simulink library "dgl_grc"  (R2024a)
settings: Solver=VariableStepAuto  StartTime=0.0  StopTime=10.0  RelTol=1e-3
undefined symbols (not defined in the file or in its folder): Diag2_bRstFault_C, Diag2_f32_UdcLowCoefAddStep_C, Diag2_f32_UdcLowCoefDepStep_C, Diag2_f32_UdcLowHysBand_C, Diag2_f32_UdcLowStartDerat_C, Diag2_f32_UdcLowStopDerat_C, Diag2_f32_UdcOverCoefAddStep_C, Diag2_f32_UdcOverCoefDepStep_C, Diag2_f32_UdcOverHysBand_C, Diag2_f32_UdcOverStartDerat_C, Diag2_f32_UdcOverStopDerat_C, Diag2_int16_HvLowErrErr_C, Diag2_int16_HvLowErrHeal_C, Diag2_int16_HvLowWarnErr_C, Diag2_int16_HvLowWarnHeal_C, Diag2_int16_HvOverErrErr_C, Diag2_int16_HvOverErrHeal_C, Diag2_int16_HvOverWarnErr_C, Diag2_int16_HvOverWarnHeal_C, DiagM_bZeroCurrMor_C, DiagM_bZeroCurrTrig_C, DiagM_Fault2LevelMor_C, DiagM_Fault2LevelTrig_C, GRC_FAKE_SAMPLE_TIME, KDGL_bBusOffEna_C, KDGL_bComInvaildVcuEna_C, KDGL_bComLostVcuEna_C, KDGL_bCurrFaultEna_C, KDGL_bEnaBenchShutDwn_C, KDGL_bEOPFaultEna_C, KDGL_bHvDcVoltFaultEna_C, KDGL_bIGNVoltFaultEna_C, KDGL_bOilTempFaultEna_C, KDGL_bPCBTempFaultEna_C, KDGL_bPosSenrFaultEna_C, KDGL_bPREREGFaultEna_C, KDGL_bRstStallPort_flg, KDGL_bSicFltFaultEna_C, KDGL_bSicTempFaultEna_C, KDGL_bTempSensrFaultEna_C, KDGL_bVCC5VFaultEna_C, KDGL_bVREF5VFaultEna_C, KDGL_bWaterTempFaultEna_C, KDGL_IGBTCoefAddStep_C, KDGL_IGBTCoefDepStep_C, KDGL_IGBTHysBand_C, KDGL_IGBTStartDerat_C, KDGL_IGBTStopDerat_C, KDGL_iMotStallProtEna_A, KDGL_MotCoefAddStep_C, KDGL_MotCoefDepStep_C, KDGL_MotHysBand_C, KDGL_MotStartDerat_C, KDGL_MotStopDerat_C, KDGL_nEOPSpdDiff_rpm, KDGL_nRotStallProtEna_rpm, KDGL_OilCoefAddStep_C, KDGL_OilCoefDepStep_C, KDGL_OilHysBand_C, KDGL_OilStartDerat_C ... (+37)
libraries: Library x28, GRC_Lib x8
(part 2 of 2)

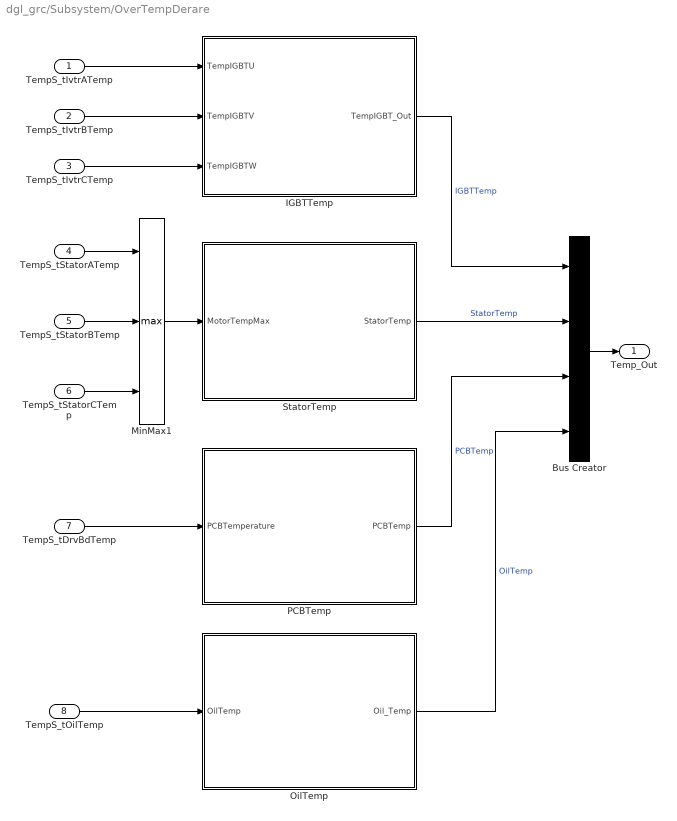
== system dgl_grc/Subsystem/OverTempDerare ==
  TempS_tIvtrATemp : Inport  OutDataTypeStr=single
  TempS_tIvtrBTemp : Inport  Port=2  OutDataTypeStr=single
  TempS_tIvtrCTemp : Inport  Port=3  OutDataTypeStr=single
  TempS_tStatorATemp : Inport  Port=4  OutDataTypeStr=single
  TempS_tStatorBTemp : Inport  Port=5  OutDataTypeStr=single
  TempS_tStatorCTemp : Inport  Port=6  OutDataTypeStr=single
  TempS_tDrvBdTemp : Inport  Port=7  OutDataTypeStr=single
  TempS_tOilTemp : Inport  Port=8  OutDataTypeStr=single
  Bus Creator : BusCreator  Inputs=4
  IGBTTemp : Subsystem
  MinMax1 : MinMax  Function=max  Inputs=3
  OilTemp : Subsystem
  PCBTemp : Subsystem
  StatorTemp : Subsystem
  Temp_Out : Outport  VectorParamsAs1DForOutWhenUnconnected=off
  wires:
  TempS_tIvtrATemp/1 -> IGBTTemp/1(TempIGBTU)
  TempS_tIvtrBTemp/1 -> IGBTTemp/2(TempIGBTV)
  TempS_tIvtrCTemp/1 -> IGBTTemp/3(TempIGBTW)
  TempS_tStatorBTemp/1 -> MinMax1/2
  TempS_tStatorATemp/1 -> MinMax1/1
  TempS_tStatorCTemp/1 -> MinMax1/3
  MinMax1/1 -> StatorTemp/1(MotorTempMax)
  TempS_tDrvBdTemp/1 -> PCBTemp/1(PCBTemperature)
  StatorTemp/1(StatorTemp) -> Bus Creator/2  "StatorTemp"
  IGBTTemp/1(TempIGBT_Out) -> Bus Creator/1  "IGBTTemp"
  PCBTemp/1(PCBTemp) -> Bus Creator/3  "PCBTemp"
  Bus Creator/1 -> Temp_Out/1
  TempS_tOilTemp/1 -> OilTemp/1(OilTemp)
  OilTemp/1(Oil_Temp) -> Bus Creator/4  "OilTemp"

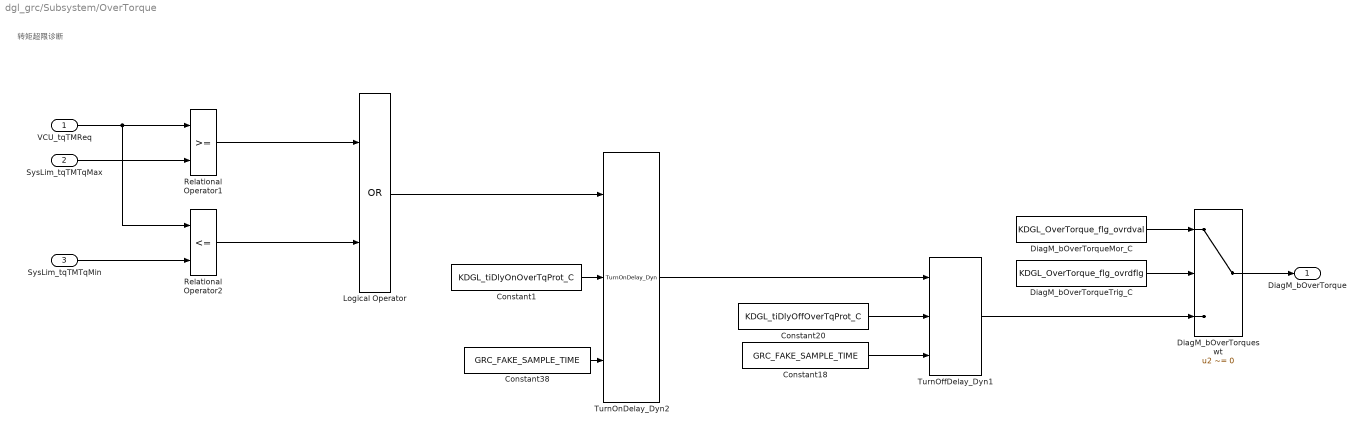
== system dgl_grc/Subsystem/OverTorque ==
  note: 转矩超限诊断
  VCU_tqTMReq : Inport  OutDataTypeStr=single
  SysLim_tqTMTqMax : Inport  Port=2  OutDataTypeStr=single
  "SysLim_tqTMTqMin " : Inport  Port=3  OutDataTypeStr=single
  Constant1 : Constant  Value=KDGL_tiDlyOnOverTqProt_C
  Constant18 : Constant  Value=GRC_FAKE_SAMPLE_TIME
  Constant20 : Constant  Value=KDGL_tiDlyOffOverTqProt_C
  Constant38 : Constant  Value=GRC_FAKE_SAMPLE_TIME
  DiagM_bOverTorqueMor_C : Constant  Value=KDGL_OverTorque_flg_ovrdval
  DiagM_bOverTorqueTrig_C : Constant  Value=KDGL_OverTorque_flg_ovrdflg
  DiagM_bOverTorqueswt : Switch  Criteria=u2 ~= 0  SaturateOnIntegerOverflow=off  InputSameDT=off
  Logical Operator : Logic  Operator=OR  AllPortsSameDT=off  OutDataTypeStr=boolean
  Relational Operator1 : RelationalOperator  OutDataTypeStr=boolean  RndMeth=Simplest  InputSameDT=off
  Relational Operator2 : RelationalOperator  Operator=<=  OutDataTypeStr=boolean  RndMeth=Simplest  InputSameDT=off
  TurnOffDelay_Dyn1 : GRC_Lib/Delay/TurnOffDelay_Dyn  IpDT=single
  TurnOnDelay_Dyn2 : GRC_Lib/Delay/TurnOnDelay_Dyn  IpDT=single
  DiagM_bOverTorque : Outport  VectorParamsAs1DForOutWhenUnconnected=off
  wires:
  Constant1/1 -> TurnOnDelay_Dyn2/2
  VCU_tqTMReq/1 -> Relational Operator2/1, Relational Operator1/1
  TurnOnDelay_Dyn2/1 -> TurnOffDelay_Dyn1/1
  Constant38/1 -> TurnOnDelay_Dyn2/3
  Constant18/1 -> TurnOffDelay_Dyn1/3
  TurnOffDelay_Dyn1/1 -> DiagM_bOverTorqueswt/3
  Constant20/1 -> TurnOffDelay_Dyn1/2
  Relational Operator1/1 -> Logical Operator/1
  SysLim_tqTMTqMax/1 -> Relational Operator1/2
  "SysLim_tqTMTqMin "/1 -> Relational Operator2/2
  Relational Operator2/1 -> Logical Operator/2
  Logical Operator/1 -> TurnOnDelay_Dyn2/1
  DiagM_bOverTorqueswt/1 -> DiagM_bOverTorque/1
  DiagM_bOverTorqueMor_C/1 -> DiagM_bOverTorqueswt/1
  DiagM_bOverTorqueTrig_C/1 -> DiagM_bOverTorqueswt/2

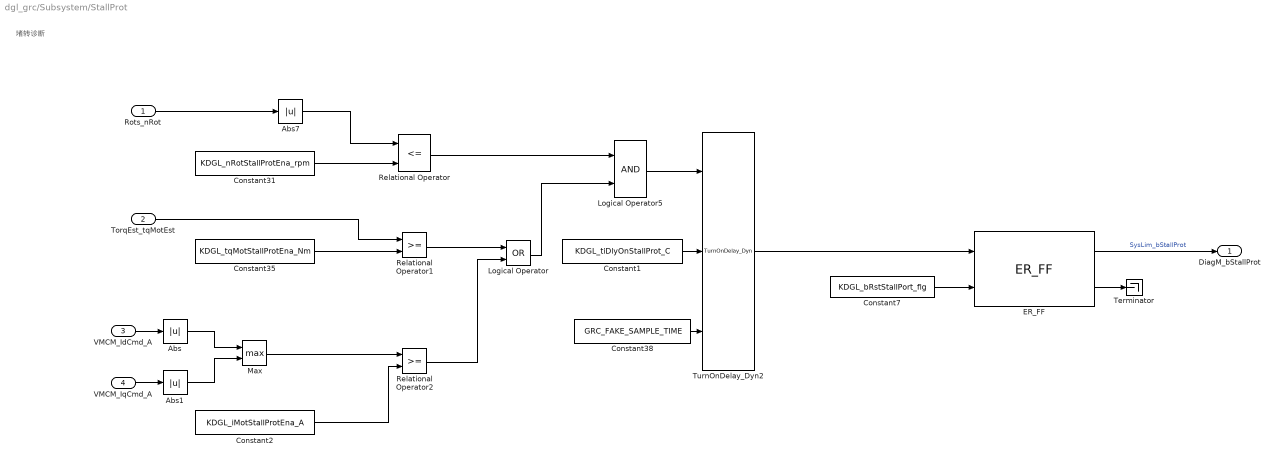
== system dgl_grc/Subsystem/StallProt ==
  note: 堵转诊断
  Rots_nRot : Inport  OutDataTypeStr=single
  TorqEst_tqMotEst : Inport  Port=2  OutDataTypeStr=single
  VMCM_IdCmd_A : Inport  Port=3  OutDataTypeStr=single
  VMCM_IqCmd_A : Inport  Port=4  OutDataTypeStr=single
  Abs : Abs  SaturateOnIntegerOverflow=off
  Abs1 : Abs  SaturateOnIntegerOverflow=off
  Abs7 : Abs  SaturateOnIntegerOverflow=off
  Constant1 : Constant  Value=KDGL_tiDlyOnStallProt_C
  Constant2 : Constant  Value=KDGL_iMotStallProtEna_A
  Constant31 : Constant  Value=KDGL_nRotStallProtEna_rpm
  Constant35 : Constant  Value=KDGL_tqMotStallProtEna_Nm
  Constant38 : Constant  Value=GRC_FAKE_SAMPLE_TIME
  Constant7 : Constant  Value=KDGL_bRstStallPort_flg
  ER_FF : GRC_Lib/Memory/ER_FF  FalseVal=0  TrueVal=1
  Logical Operator : Logic  Operator=OR  AllPortsSameDT=off  OutDataTypeStr=boolean
  Logical Operator5 : Logic  AllPortsSameDT=off  OutDataTypeStr=boolean
  Max : MinMax  Function=max  Inputs=2
  Relational Operator : RelationalOperator  Operator=<=  OutDataTypeStr=boolean  RndMeth=Simplest  InputSameDT=off
  Relational Operator1 : RelationalOperator  OutDataTypeStr=boolean  RndMeth=Simplest  InputSameDT=off
  Relational Operator2 : RelationalOperator  OutDataTypeStr=boolean  RndMeth=Simplest  InputSameDT=off
  Terminator : Terminator
  TurnOnDelay_Dyn2 : GRC_Lib/Delay/TurnOnDelay_Dyn  IpDT=single
  DiagM_bStallProt : Outport  VectorParamsAs1DForOutWhenUnconnected=off
  wires:
  ER_FF/1 -> DiagM_bStallProt/1  "SysLim_bStallProt"
  Abs7/1 -> Relational Operator/1
  Rots_nRot/1 -> Abs7/1
  Logical Operator5/1 -> TurnOnDelay_Dyn2/1
  Constant35/1 -> Relational Operator1/2
  Relational Operator/1 -> Logical Operator5/1
  Relational Operator1/1 -> Logical Operator/1
  Constant38/1 -> TurnOnDelay_Dyn2/3
  Constant31/1 -> Relational Operator/2
  TorqEst_tqMotEst/1 -> Relational Operator1/1
  Constant1/1 -> TurnOnDelay_Dyn2/2
  TurnOnDelay_Dyn2/1 -> ER_FF/1
  Constant7/1 -> ER_FF/2
  ER_FF/2 -> Terminator/1
  VMCM_IdCmd_A/1 -> Abs/1
  VMCM_IqCmd_A/1 -> Abs1/1
  Abs/1 -> Max/1
  Abs1/1 -> Max/2
  Max/1 -> Relational Operator2/1
  Constant2/1 -> Relational Operator2/2
  Relational Operator2/1 -> Logical Operator/2
  Logical Operator/1 -> Logical Operator5/2

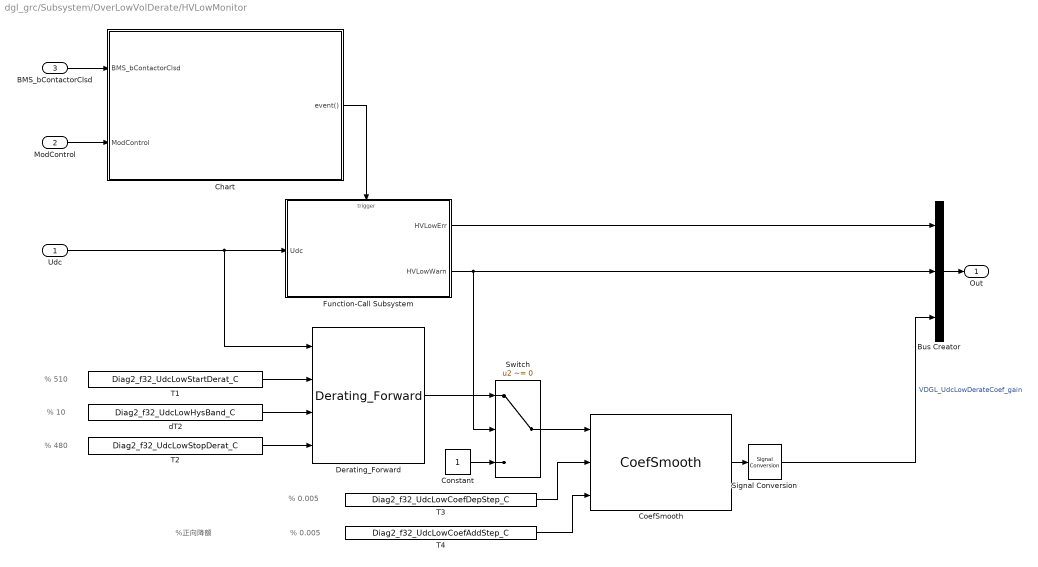
== system dgl_grc/Subsystem/OverLowVolDerate/HVLowMonitor ==
  note: % 510
  note: % 0.005
  note: %正向降额
  note: % 0.005
  note: % 480
  note: % 10
  Udc : Inport
  ModControl : Inport  Port=2
  BMS_bContactorClsd : Inport  Port=3
  Bus Creator : BusCreator  Inputs=3
  Chart : Stateflow chart  TreatAsAtomicUnit=on
  CoefSmooth : Library/CoefSmooth  SystemSampleTime=-1  VariantActivationTime=update diagram  AllowFlexibleInterface=on  Latency=0  AutoFrameSizeCalculation=off
  Constant : Constant  OutDataTypeStr=single
  Derating_Forward : Library/Derating_Forward  SystemSampleTime=-1  VariantActivationTime=update diagram  AllowFlexibleInterface=on  Latency=0  AutoFrameSizeCalculation=off
  Function-Call Subsystem : Subsystem  TreatAsAtomicUnit=on
  Signal Conversion : SignalConversion  OverrideOpt=off
  Switch : Switch  Criteria=u2 ~= 0  SaturateOnIntegerOverflow=off  InputSameDT=off
  T1 : Constant  Value=Diag2_f32_UdcLowStartDerat_C  OutDataTypeStr=single
  T2 : Constant  Value=Diag2_f32_UdcLowStopDerat_C  OutDataTypeStr=single
  T3 : Constant  Value=Diag2_f32_UdcLowCoefDepStep_C  OutDataTypeStr=single
  T4 : Constant  Value=Diag2_f32_UdcLowCoefAddStep_C  OutDataTypeStr=single
  dT2 : Constant  Value=Diag2_f32_UdcLowHysBand_C  OutDataTypeStr=single
  Out : Outport  VectorParamsAs1DForOutWhenUnconnected=off
  wires:
  Chart/1(event()) -> Function-Call Subsystem/Trigger
  Function-Call Subsystem/1(HVLowErr) -> Bus Creator/1
  Bus Creator/1 -> Out/1
  Function-Call Subsystem/2(HVLowWarn) -> Switch/2, Bus Creator/2
  dT2/1 -> Derating_Forward/3
  T1/1 -> Derating_Forward/2
  T2/1 -> Derating_Forward/4
  Derating_Forward/1 -> Switch/1
  Constant/1 -> Switch/3
  Switch/1 -> CoefSmooth/1
  T3/1 -> CoefSmooth/2
  T4/1 -> CoefSmooth/3
  CoefSmooth/1 -> Signal Conversion/1
  Signal Conversion/1 -> Bus Creator/3  "VDGL_UdcLowDerateCoef_gain"
  ModControl/1 -> Chart/2(ModControl)
  Udc/1 -> Derating_Forward/1, Function-Call Subsystem/1(Udc)
  BMS_bContactorClsd/1 -> Chart/1(BMS_bContactorClsd)

== system dgl_grc/Subsystem/OverLowVolDerate/HVOverMonitor ==
  note: 反向降额
  note: % 20
  note: % 880
  note: % 750
  note: % 0.005
  note: % 0.005
  Udc : Inport
  Bus Creator : BusCreator  Inputs=3
  CoefSmooth : Library/CoefSmooth  SystemSampleTime=-1  VariantActivationTime=update diagram  AllowFlexibleInterface=on  Latency=0  AutoFrameSizeCalculation=off
  Constant : Constant  OutDataTypeStr=single
  Derating_Reverse : Library/Derating_Reverse  SystemSampleTime=-1  VariantActivationTime=update diagram  AllowFlexibleInterface=on  Latency=0  AutoFrameSizeCalculation=off
  Function-Call Subsystem : Subsystem  TreatAsAtomicUnit=on
  Signal Conversion : SignalConversion  OverrideOpt=off
  Switch : Switch  Criteria=u2 ~= 0  SaturateOnIntegerOverflow=off  InputSameDT=off
  T1 : Constant  Value=Diag2_f32_UdcOverStartDerat_C  OutDataTypeStr=single
  T2 : Constant  Value=Diag2_f32_UdcOverStopDerat_C  OutDataTypeStr=single
  T3 : Constant  Value=Diag2_f32_UdcOverCoefDepStep_C  OutDataTypeStr=single
  T4 : Constant  Value=Diag2_f32_UdcOverCoefAddStep_C  OutDataTypeStr=single
  dT2 : Constant  Value=Diag2_f32_UdcOverHysBand_C  OutDataTypeStr=single
  Out : Outport  VectorParamsAs1DForOutWhenUnconnected=off
  wires:
  Udc/1 -> Derating_Reverse/1, Function-Call Subsystem/1(Udc)
  Bus Creator/1 -> Out/1
  Function-Call Subsystem/2(HVOverWarn) -> Switch/2, Bus Creator/2
  Function-Call Subsystem/1(HVOverErr) -> Bus Creator/1
  dT2/1 -> Derating_Reverse/3
  T1/1 -> Derating_Reverse/2
  T2/1 -> Derating_Reverse/4
  Derating_Reverse/1 -> Switch/1
  Constant/1 -> Switch/3
  Switch/1 -> CoefSmooth/1
  T3/1 -> CoefSmooth/2
  T4/1 -> CoefSmooth/3
  CoefSmooth/1 -> Signal Conversion/1
  Signal Conversion/1 -> Bus Creator/3  "VDGL_UdcOverDerateCoef_gain"

== system dgl_grc/Subsystem/OverSpdDerate/Function-Call Subsystem ==
  note: % 20
  note: % -20
  note: % 1000
  note: % 22000
  note: %速度滞环
  MeclSpd : Inport
  Constant : Constant  Value=KDGL_OverSpd_rpm  OutDataTypeStr=single
  Constant1 : Constant  Value=KDGL_OverSpdHeal_cnt  OutDataTypeStr=int16
  Constant2 : Constant  Value=KDGL_OverSpdErr_cnt  OutDataTypeStr=int16
  Constant3 : Constant  Value=KDGL_OverSpdHysBand_rpm  OutDataTypeStr=single
  Hysteresis_Ctrl_Forward : Library/Hysteresis_Ctrl_Forward  SystemSampleTime=-1  VariantActivationTime=update diagram  AllowFlexibleInterface=on  Latency=0  AutoFrameSizeCalculation=off
  Signal Conversion : SignalConversion  OverrideOpt=off
  debounce : Library/debounce  SystemSampleTime=-1  VariantActivationTime=update diagram  AllowFlexibleInterface=on  Latency=0  AutoFrameSizeCalculation=off
  OverSpdFlg : Outport  VectorParamsAs1DForOutWhenUnconnected=off
  wires:
  Constant1/1 -> debounce/2
  Constant2/1 -> debounce/3
  Signal Conversion/1 -> OverSpdFlg/1
  debounce/1 -> Signal Conversion/1
  Constant/1 -> Hysteresis_Ctrl_Forward/2
  Constant3/1 -> Hysteresis_Ctrl_Forward/3
  Hysteresis_Ctrl_Forward/1 -> debounce/1
  MeclSpd/1 -> Hysteresis_Ctrl_Forward/1

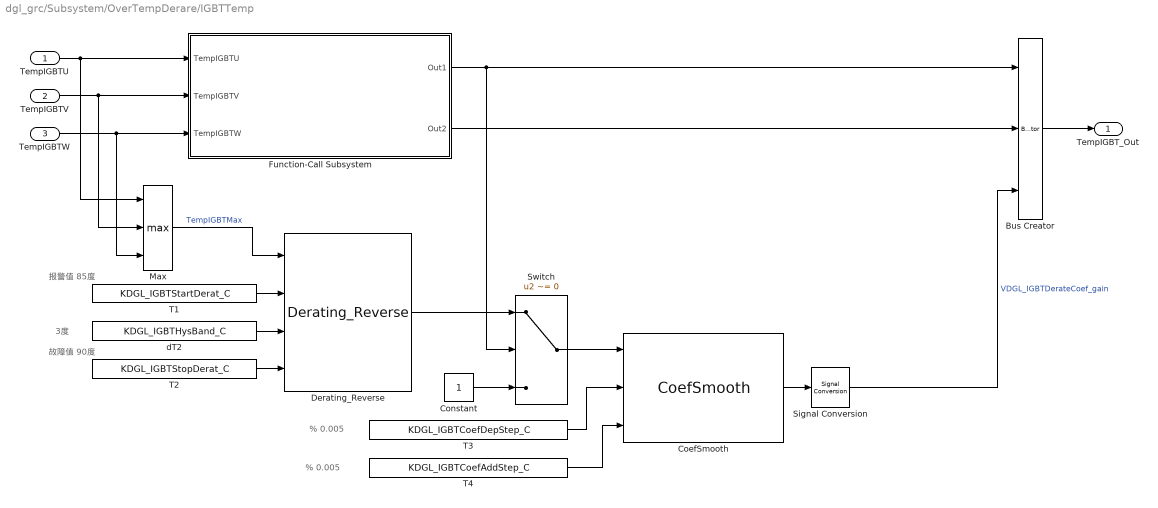
== system dgl_grc/Subsystem/OverTempDerare/IGBTTemp ==
  note: % 0.005
  note: 报警值
      | 85度
  note: 3度
  note: 故障值
      | 90度
  note: % 0.005
  TempIGBTU : Inport
  TempIGBTV : Inport  Port=2
  TempIGBTW : Inport  Port=3
  Bus Creator : BusCreator  Inputs=3
  CoefSmooth : Library/CoefSmooth  SystemSampleTime=-1  VariantActivationTime=update diagram  AllowFlexibleInterface=on  Latency=0  AutoFrameSizeCalculation=off
  Constant : Constant  OutDataTypeStr=single
  Derating_Reverse : Library/Derating_Reverse  SystemSampleTime=-1  VariantActivationTime=update diagram  AllowFlexibleInterface=on  Latency=0  AutoFrameSizeCalculation=off
  Function-Call Subsystem : Subsystem  TreatAsAtomicUnit=on
  Max : MinMax  Function=max  Inputs=3
  Signal Conversion : SignalConversion  OverrideOpt=off
  Switch : Switch  Criteria=u2 ~= 0  SaturateOnIntegerOverflow=off  InputSameDT=off
  T1 : Constant  Value=KDGL_IGBTStartDerat_C  OutDataTypeStr=single
  T2 : Constant  Value=KDGL_IGBTStopDerat_C  OutDataTypeStr=single
  T3 : Constant  Value=KDGL_IGBTCoefDepStep_C  OutDataTypeStr=single
  T4 : Constant  Value=KDGL_IGBTCoefAddStep_C  OutDataTypeStr=single
  dT2 : Constant  Value=KDGL_IGBTHysBand_C  OutDataTypeStr=single
  TempIGBT_Out : Outport  VectorParamsAs1DForOutWhenUnconnected=off
  wires:
  Bus Creator/1 -> TempIGBT_Out/1
  Function-Call Subsystem/1(Out1) -> Switch/2, Bus Creator/1
  Function-Call Subsystem/2(Out2) -> Bus Creator/2
  dT2/1 -> Derating_Reverse/3
  T1/1 -> Derating_Reverse/2
  T2/1 -> Derating_Reverse/4
  Derating_Reverse/1 -> Switch/1
  Constant/1 -> Switch/3
  Switch/1 -> CoefSmooth/1
  T3/1 -> CoefSmooth/2
  T4/1 -> CoefSmooth/3
  CoefSmooth/1 -> Signal Conversion/1
  Signal Conversion/1 -> Bus Creator/3  "VDGL_IGBTDerateCoef_gain"
  TempIGBTU/1 -> Max/1, Function-Call Subsystem/1(TempIGBTU)
  TempIGBTV/1 -> Max/2, Function-Call Subsystem/2(TempIGBTV)
  TempIGBTW/1 -> Max/3, Function-Call Subsystem/3(TempIGBTW)
  Max/1 -> Derating_Reverse/1  "TempIGBTMax"

== system dgl_grc/Subsystem/OverTempDerare/OilTemp ==
  note: % 0.005
  note: 报警值
      | 110度
  note: 3度
  note: 故障值
      | 120度
  note: % 0.005
  OilTemp : Inport
  Bus Creator : BusCreator  Inputs=3
  CoefSmooth : Library/CoefSmooth  SystemSampleTime=-1  VariantActivationTime=update diagram  AllowFlexibleInterface=on  Latency=0  AutoFrameSizeCalculation=off
  Constant : Constant  OutDataTypeStr=single
  Derating_Reverse : Library/Derating_Reverse  SystemSampleTime=-1  VariantActivationTime=update diagram  AllowFlexibleInterface=on  Latency=0  AutoFrameSizeCalculation=off
  Function-Call Subsystem : Subsystem  TreatAsAtomicUnit=on
  Signal Conversion : SignalConversion  OverrideOpt=off
  Switch : Switch  Criteria=u2 ~= 0  SaturateOnIntegerOverflow=off  InputSameDT=off
  T1 : Constant  Value=KDGL_OilStartDerat_C  OutDataTypeStr=single
  T2 : Constant  Value=KDGL_OilStopDerat_C  OutDataTypeStr=single
  T3 : Constant  Value=KDGL_OilCoefDepStep_C  OutDataTypeStr=single
  T4 : Constant  Value=KDGL_OilCoefAddStep_C  OutDataTypeStr=single
  dT2 : Constant  Value=KDGL_OilHysBand_C  OutDataTypeStr=single
  Oil_Temp : Outport  VectorParamsAs1DForOutWhenUnconnected=off
  wires:
  Bus Creator/1 -> Oil_Temp/1
  Function-Call Subsystem/2(Out1) -> Bus Creator/2
  Function-Call Subsystem/1(Out) -> Switch/2, Bus Creator/1
  dT2/1 -> Derating_Reverse/3
  T1/1 -> Derating_Reverse/2
  T2/1 -> Derating_Reverse/4
  Derating_Reverse/1 -> Switch/1
  Constant/1 -> Switch/3
  Switch/1 -> CoefSmooth/1
  T3/1 -> CoefSmooth/2
  T4/1 -> CoefSmooth/3
  CoefSmooth/1 -> Signal Conversion/1
  Signal Conversion/1 -> Bus Creator/3  "VDGL_OilDerateCoef_gain"
  OilTemp/1 -> Derating_Reverse/1, Function-Call Subsystem/1(OilTemp)

== system dgl_grc/Subsystem/OverTempDerare/PCBTemp ==
  note: 报警值
      | 85度
  note: 3度
  note: 故障值
      | 90度
  note: % 0.005
  note: % 0.005
  PCBTemperature : Inport
  Bus Creator : BusCreator  Inputs=3
  CoefSmooth : Library/CoefSmooth  SystemSampleTime=-1  VariantActivationTime=update diagram  AllowFlexibleInterface=on  Latency=0  AutoFrameSizeCalculation=off
  Constant : Constant  OutDataTypeStr=single
  Derating_Reverse : Library/Derating_Reverse  SystemSampleTime=-1  VariantActivationTime=update diagram  AllowFlexibleInterface=on  Latency=0  AutoFrameSizeCalculation=off
  Function-Call Subsystem : Subsystem  TreatAsAtomicUnit=on
  Signal Conversion : SignalConversion  OverrideOpt=off
  Switch : Switch  Criteria=u2 ~= 0  SaturateOnIntegerOverflow=off  InputSameDT=off
  T1 : Constant  Value=KDGL_PCBStartDerat_C  OutDataTypeStr=single
  T2 : Constant  Value=KDGL_PCBStopDerat_C  OutDataTypeStr=single
  T3 : Constant  Value=KDGL_PCBCoefDepStep_C  OutDataTypeStr=single
  T4 : Constant  Value=KDGL_PCBCoefAddStep_C  OutDataTypeStr=single
  dT2 : Constant  Value=KDGL_PCBHysBand_C  OutDataTypeStr=single
  PCBTemp : Outport  VectorParamsAs1DForOutWhenUnconnected=off
  wires:
  Bus Creator/1 -> PCBTemp/1
  Function-Call Subsystem/2(Out1) -> Bus Creator/2
  Function-Call Subsystem/1(Out) -> Switch/2, Bus Creator/1
  dT2/1 -> Derating_Reverse/3
  T1/1 -> Derating_Reverse/2
  T2/1 -> Derating_Reverse/4
  Derating_Reverse/1 -> Switch/1
  Constant/1 -> Switch/3
  Switch/1 -> CoefSmooth/1
  T3/1 -> CoefSmooth/2
  T4/1 -> CoefSmooth/3
  CoefSmooth/1 -> Signal Conversion/1
  Signal Conversion/1 -> Bus Creator/3  "VDGL_PCBDerateCoef_gain"
  PCBTemperature/1 -> Derating_Reverse/1, Function-Call Subsystem/1(PCBTemp)

== system dgl_grc/Subsystem/OverTempDerare/StatorTemp ==
  note: 10度
  note: 故障值
      | 120度
  note: 报警值
      | 110度
  note: % 0.005
  note: % 0.005
  MotorTempMax : Inport
  Bus Creator : BusCreator  Inputs=3
  CoefSmooth : Library/CoefSmooth  SystemSampleTime=-1  VariantActivationTime=update diagram  AllowFlexibleInterface=on  Latency=0  AutoFrameSizeCalculation=off
  Constant : Constant  OutDataTypeStr=single
  Function-Call Subsystem : Subsystem  TreatAsAtomicUnit=on
  Signal Conversion : SignalConversion  OverrideOpt=off
  Switch : Switch  Criteria=u2 ~= 0  SaturateOnIntegerOverflow=off  InputSameDT=off
  T3 : Constant  Value=KDGL_MotStartDerat_C  OutDataTypeStr=single
  T4 : Constant  Value=KDGL_MotStopDerat_C  OutDataTypeStr=single
  T5 : Constant  Value=KDGL_MotCoefDepStep_C  OutDataTypeStr=single
  T6 : Constant  Value=KDGL_MotCoefAddStep_C  OutDataTypeStr=single
  Temp_Derating_Reverse : Library/Derating_Reverse  SystemSampleTime=-1  VariantActivationTime=update diagram  AllowFlexibleInterface=on  Latency=0  AutoFrameSizeCalculation=off
  dT1 : Constant  Value=KDGL_MotHysBand_C  OutDataTypeStr=single
  StatorTemp : Outport  VectorParamsAs1DForOutWhenUnconnected=off
  wires:
  MotorTempMax/1 -> Temp_Derating_Reverse/1, Function-Call Subsystem/1(MotorTemp)
  Bus Creator/1 -> StatorTemp/1
  Function-Call Subsystem/2(Out2) -> Bus Creator/2
  dT1/1 -> Temp_Derating_Reverse/3
  T3/1 -> Temp_Derating_Reverse/2
  T4/1 -> Temp_Derating_Reverse/4
  Function-Call Subsystem/1(Out1) -> Switch/2, Bus Creator/1
  Temp_Derating_Reverse/1 -> Switch/1
  Constant/1 -> Switch/3
  Switch/1 -> CoefSmooth/1
  T5/1 -> CoefSmooth/2
  T6/1 -> CoefSmooth/3
  CoefSmooth/1 -> Signal Conversion/1
  Signal Conversion/1 -> Bus Creator/3  "VDGL_MotDerateCoef_gain"

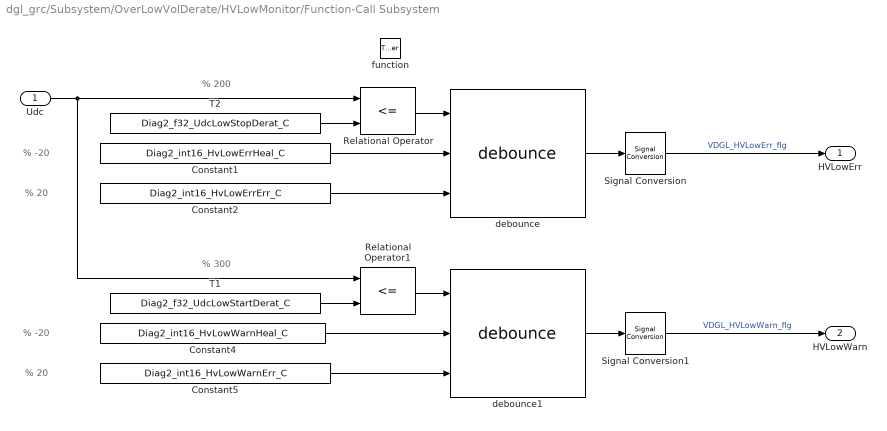
== system dgl_grc/Subsystem/OverLowVolDerate/HVLowMonitor/Function-Call Subsystem ==
  note: % 20
  note: % -20
  note: % 200
  note: % 300
  note: % 20
  note: % -20
  Udc : Inport
  function : TriggerPort  TriggerType=function-call  VariantControl=(inherit)
  Constant1 : Constant  Value=Diag2_int16_HvLowErrHeal_C  OutDataTypeStr=int16
  Constant2 : Constant  Value=Diag2_int16_HvLowErrErr_C  OutDataTypeStr=int16
  Constant4 : Constant  Value=Diag2_int16_HvLowWarnHeal_C  OutDataTypeStr=int16
  Constant5 : Constant  Value=Diag2_int16_HvLowWarnErr_C  OutDataTypeStr=int16
  Relational Operator : RelationalOperator  Operator=<=  OutDataTypeStr=boolean  InputSameDT=off
  Relational Operator1 : RelationalOperator  Operator=<=  OutDataTypeStr=boolean  InputSameDT=off
  Signal Conversion : SignalConversion  OverrideOpt=off
  Signal Conversion1 : SignalConversion  OverrideOpt=off
  T1 : Constant  Value=Diag2_f32_UdcLowStartDerat_C  OutDataTypeStr=single
  T2 : Constant  Value=Diag2_f32_UdcLowStopDerat_C  OutDataTypeStr=single
  debounce : Library/debounce  SystemSampleTime=-1  VariantActivationTime=update diagram  AllowFlexibleInterface=on  Latency=0  AutoFrameSizeCalculation=off
  debounce1 : Library/debounce  SystemSampleTime=-1  VariantActivationTime=update diagram  AllowFlexibleInterface=on  Latency=0  AutoFrameSizeCalculation=off
  HVLowErr : Outport  VectorParamsAs1DForOutWhenUnconnected=off
  HVLowWarn : Outport  Port=2  VectorParamsAs1DForOutWhenUnconnected=off
  wires:
  Udc/1 -> Relational Operator1/1, Relational Operator/1
  T2/1 -> Relational Operator/2
  Relational Operator/1 -> debounce/1
  Constant1/1 -> debounce/2
  Constant2/1 -> debounce/3
  Signal Conversion/1 -> HVLowErr/1  "VDGL_HVLowErr_flg"
  debounce/1 -> Signal Conversion/1
  T1/1 -> Relational Operator1/2
  Relational Operator1/1 -> debounce1/1
  Constant4/1 -> debounce1/2
  Constant5/1 -> debounce1/3
  Signal Conversion1/1 -> HVLowWarn/1  "VDGL_HVLowWarn_flg"
  debounce1/1 -> Signal Conversion1/1

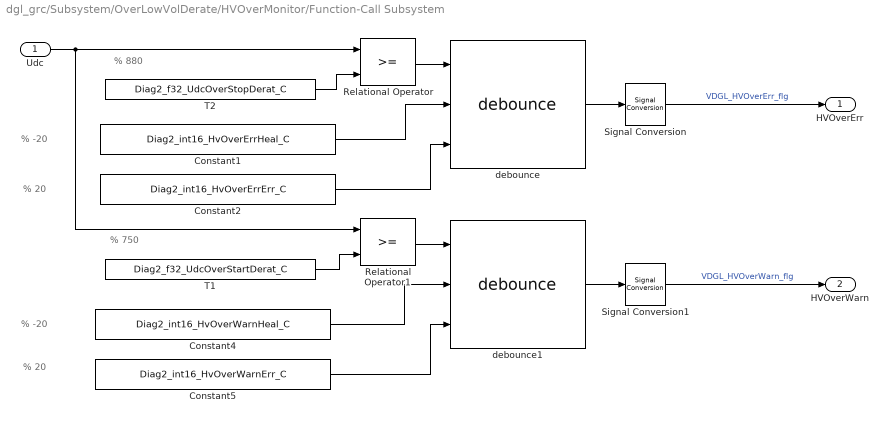
== system dgl_grc/Subsystem/OverLowVolDerate/HVOverMonitor/Function-Call Subsystem ==
  note: % 750
  note: % 880
  note: % 20
  note: % -20
  note: % 20
  note: % -20
  Udc : Inport
  Constant1 : Constant  Value=Diag2_int16_HvOverErrHeal_C  OutDataTypeStr=int16
  Constant2 : Constant  Value=Diag2_int16_HvOverErrErr_C  OutDataTypeStr=int16
  Constant4 : Constant  Value=Diag2_int16_HvOverWarnHeal_C  OutDataTypeStr=int16
  Constant5 : Constant  Value=Diag2_int16_HvOverWarnErr_C  OutDataTypeStr=int16
  Relational Operator : RelationalOperator  OutDataTypeStr=boolean  InputSameDT=off
  Relational Operator1 : RelationalOperator  OutDataTypeStr=boolean  InputSameDT=off
  Signal Conversion : SignalConversion  OverrideOpt=off
  Signal Conversion1 : SignalConversion  OverrideOpt=off
  T1 : Constant  Value=Diag2_f32_UdcOverStartDerat_C  OutDataTypeStr=single
  T2 : Constant  Value=Diag2_f32_UdcOverStopDerat_C  OutDataTypeStr=single
  debounce : Library/debounce  SystemSampleTime=-1  VariantActivationTime=update diagram  AllowFlexibleInterface=on  Latency=0  AutoFrameSizeCalculation=off
  debounce1 : Library/debounce  SystemSampleTime=-1  VariantActivationTime=update diagram  AllowFlexibleInterface=on  Latency=0  AutoFrameSizeCalculation=off
  HVOverErr : Outport  VectorParamsAs1DForOutWhenUnconnected=off
  HVOverWarn : Outport  Port=2  VectorParamsAs1DForOutWhenUnconnected=off
  wires:
  Udc/1 -> Relational Operator1/1, Relational Operator/1
  T2/1 -> Relational Operator/2
  Relational Operator/1 -> debounce/1
  Constant1/1 -> debounce/2
  Constant2/1 -> debounce/3
  Signal Conversion/1 -> HVOverErr/1  "VDGL_HVOverErr_flg"
  debounce/1 -> Signal Conversion/1
  T1/1 -> Relational Operator1/2
  Relational Operator1/1 -> debounce1/1
  Constant4/1 -> debounce1/2
  Constant5/1 -> debounce1/3
  Signal Conversion1/1 -> HVOverWarn/1  "VDGL_HVOverWarn_flg"
  debounce1/1 -> Signal Conversion1/1

== system dgl_grc/Subsystem/OverTempDerare/IGBTTemp/Function-Call Subsystem ==
  TempIGBTU : Inport
  TempIGBTV : Inport  Port=2
  TempIGBTW : Inport  Port=3
  IGBTTempFault : Subsystem
  IGBTTempWarning : Subsystem
  Out1 : Outport  VectorParamsAs1DForOutWhenUnconnected=off
  Out2 : Outport  Port=2  VectorParamsAs1DForOutWhenUnconnected=off
  wires:
  TempIGBTU/1 -> IGBTTempWarning/1(In1), IGBTTempFault/1(In1)
  TempIGBTV/1 -> IGBTTempWarning/2(In2), IGBTTempFault/2(In2)
  TempIGBTW/1 -> IGBTTempFault/3(In3), IGBTTempWarning/3(In3)
  IGBTTempWarning/1(Out1) -> Out1/1  "VDGL_TempIGBTWarning_flg"
  IGBTTempFault/1(Out) -> Out2/1  "VDGL_TempIGBTFault_flg"

== system dgl_grc/Subsystem/OverTempDerare/OilTemp/Function-Call Subsystem ==
  note: 报警值
      | 110度
  note: 故障值
      | 120度
  note: % 20
  note: % -20
  note: % 20
  note: % -20
  OilTemp : Inport
  Constant1 : Constant  Value=KDGL_TempOilWarningHeal_C  OutDataTypeStr=int16
  Constant2 : Constant  Value=KDGL_TempOilWarningErr_C  OutDataTypeStr=int16
  Constant4 : Constant  Value=KDGL_TempOilFaultHeal_C  OutDataTypeStr=int16
  Constant5 : Constant  Value=KDGL_TempOilFaultErr_C  OutDataTypeStr=int16
  Relational Operator : RelationalOperator  OutDataTypeStr=boolean  InputSameDT=off
  Relational Operator1 : RelationalOperator  OutDataTypeStr=boolean  InputSameDT=off
  Signal Conversion : SignalConversion  OverrideOpt=off
  Signal Conversion1 : SignalConversion  OverrideOpt=off
  T1 : Constant  Value=KDGL_OilStartDerat_C  OutDataTypeStr=single
  T2 : Constant  Value=KDGL_OilStopDerat_C  OutDataTypeStr=single
  debounce : Library/debounce  SystemSampleTime=-1  VariantActivationTime=update diagram  AllowFlexibleInterface=on  Latency=0  AutoFrameSizeCalculation=off
  debounce1 : Library/debounce  SystemSampleTime=-1  VariantActivationTime=update diagram  AllowFlexibleInterface=on  Latency=0  AutoFrameSizeCalculation=off
  Out : Outport  VectorParamsAs1DForOutWhenUnconnected=off
  Out1 : Outport  Port=2  VectorParamsAs1DForOutWhenUnconnected=off
  wires:
  OilTemp/1 -> Relational Operator1/1, Relational Operator/1
  T1/1 -> Relational Operator/2
  Relational Operator/1 -> debounce/1
  Constant1/1 -> debounce/2
  Constant2/1 -> debounce/3
  Signal Conversion/1 -> Out/1  "VDGL_TempOilWarning_flg"
  debounce/1 -> Signal Conversion/1
  T2/1 -> Relational Operator1/2
  Relational Operator1/1 -> debounce1/1
  Constant4/1 -> debounce1/2
  Constant5/1 -> debounce1/3
  Signal Conversion1/1 -> Out1/1  "VDGL_TempOilFault_flg"
  debounce1/1 -> Signal Conversion1/1

== system dgl_grc/Subsystem/OverTempDerare/PCBTemp/Function-Call Subsystem ==
  note: 报警值
      | 85度
  note: 故障值
      | 90度
  note: % 20
  note: % -20
  note: % 20
  note: % -20
  PCBTemp : Inport
  Constant1 : Constant  Value=KDGL_TempPCBWarningHeal_C  OutDataTypeStr=int16
  Constant2 : Constant  Value=KDGL_TempPCBWarningErr_C  OutDataTypeStr=int16
  Constant4 : Constant  Value=KDGL_TempPCBFaultHeal_C  OutDataTypeStr=int16
  Constant5 : Constant  Value=KDGL_TempPCBFaultErr_C  OutDataTypeStr=int16
  Relational Operator : RelationalOperator  OutDataTypeStr=boolean  InputSameDT=off
  Relational Operator1 : RelationalOperator  OutDataTypeStr=boolean  InputSameDT=off
  Signal Conversion : SignalConversion  OverrideOpt=off
  Signal Conversion1 : SignalConversion  OverrideOpt=off
  T1 : Constant  Value=KDGL_PCBStartDerat_C  OutDataTypeStr=single
  T2 : Constant  Value=KDGL_PCBStopDerat_C  OutDataTypeStr=single
  debounce : Library/debounce  SystemSampleTime=-1  VariantActivationTime=update diagram  AllowFlexibleInterface=on  Latency=0  AutoFrameSizeCalculation=off
  debounce1 : Library/debounce  SystemSampleTime=-1  VariantActivationTime=update diagram  AllowFlexibleInterface=on  Latency=0  AutoFrameSizeCalculation=off
  Out : Outport  VectorParamsAs1DForOutWhenUnconnected=off
  Out1 : Outport  Port=2  VectorParamsAs1DForOutWhenUnconnected=off
  wires:
  PCBTemp/1 -> Relational Operator1/1, Relational Operator/1
  T1/1 -> Relational Operator/2
  Relational Operator/1 -> debounce/1
  Constant1/1 -> debounce/2
  Constant2/1 -> debounce/3
  Signal Conversion/1 -> Out/1  "VDGL_TempPCBWarning_flg"
  debounce/1 -> Signal Conversion/1
  T2/1 -> Relational Operator1/2
  Relational Operator1/1 -> debounce1/1
  Constant4/1 -> debounce1/2
  Constant5/1 -> debounce1/3
  Signal Conversion1/1 -> Out1/1  "VDGL_TempPCBFault_flg"
  debounce1/1 -> Signal Conversion1/1

== system dgl_grc/Subsystem/OverTempDerare/StatorTemp/Function-Call Subsystem ==
  note: 120度
  note: 110度
  note: % 20
  note: % -20
  note: % 20
  note: % -20
  MotorTemp : Inport
  Constant1 : Constant  Value=KDGL_TempMotWarningHeal_C  OutDataTypeStr=int16
  Constant2 : Constant  Value=KDGL_TempMotWarningErr_C  OutDataTypeStr=int16
  Constant4 : Constant  Value=KDGL_TempMotFaultHeal_C  OutDataTypeStr=int16
  Constant5 : Constant  Value=KDGL_TempMotFaultErr_C  OutDataTypeStr=int16
  Relational Operator : RelationalOperator  OutDataTypeStr=boolean  InputSameDT=off
  Relational Operator1 : RelationalOperator  OutDataTypeStr=boolean  InputSameDT=off
  Signal Conversion : SignalConversion  OverrideOpt=off
  Signal Conversion1 : SignalConversion  OverrideOpt=off
  T3 : Constant  Value=KDGL_MotStartDerat_C  OutDataTypeStr=single
  T4 : Constant  Value=KDGL_MotStopDerat_C  OutDataTypeStr=single
  debounce : Library/debounce  SystemSampleTime=-1  VariantActivationTime=update diagram  AllowFlexibleInterface=on  Latency=0  AutoFrameSizeCalculation=off
  debounce1 : Library/debounce  SystemSampleTime=-1  VariantActivationTime=update diagram  AllowFlexibleInterface=on  Latency=0  AutoFrameSizeCalculation=off
  Out1 : Outport  VectorParamsAs1DForOutWhenUnconnected=off
  Out2 : Outport  Port=2  VectorParamsAs1DForOutWhenUnconnected=off
  wires:
  T3/1 -> Relational Operator/2
  Relational Operator/1 -> debounce/1
  Constant1/1 -> debounce/2
  Constant2/1 -> debounce/3
  Signal Conversion/1 -> Out1/1  "VDGL_TempMotWarning_flg"
  debounce/1 -> Signal Conversion/1
  T4/1 -> Relational Operator1/2
  Relational Operator1/1 -> debounce1/1
  Constant4/1 -> debounce1/2
  Constant5/1 -> debounce1/3
  debounce1/1 -> Signal Conversion1/1
  MotorTemp/1 -> Relational Operator1/1, Relational Operator/1
  Signal Conversion1/1 -> Out2/1  "VDGL_TempMotFault_flg"

== system dgl_grc/Subsystem/OverTempDerare/IGBTTemp/Function-Call Subsystem/IGBTTempFault ==
  note: % 90
  note: % 20
  note: % -20
  In1 : Inport
  In2 : Inport  Port=2
  In3 : Inport  Port=3
  Constant1 : Constant  Value=KDGL_TempIGBTFaultHeal_C  OutDataTypeStr=int16
  Constant2 : Constant  Value=KDGL_TempIGBTFaultErr_C  OutDataTypeStr=int16
  Logical Operator : Logic  Operator=OR  Inputs=3  AllPortsSameDT=off  OutDataTypeStr=boolean
  Relational Operator : RelationalOperator  OutDataTypeStr=boolean  InputSameDT=off
  Relational Operator1 : RelationalOperator  OutDataTypeStr=boolean  InputSameDT=off
  Relational Operator2 : RelationalOperator  OutDataTypeStr=boolean  InputSameDT=off
  Signal Conversion : SignalConversion  OverrideOpt=off
  T2 : Constant  Value=KDGL_IGBTStopDerat_C  OutDataTypeStr=single
  debounce : Library/debounce  SystemSampleTime=-1  VariantActivationTime=update diagram  AllowFlexibleInterface=on  Latency=0  AutoFrameSizeCalculation=off
  Out : Outport  VectorParamsAs1DForOutWhenUnconnected=off
  wires:
  In1/1 -> Relational Operator/1
  T2/1 -> Relational Operator2/2, Relational Operator1/2, Relational Operator/2
  In2/1 -> Relational Operator1/1
  In3/1 -> Relational Operator2/1
  Constant1/1 -> debounce/2
  Constant2/1 -> debounce/3
  Relational Operator/1 -> Logical Operator/1
  Relational Operator2/1 -> Logical Operator/3
  Relational Operator1/1 -> Logical Operator/2
  Logical Operator/1 -> debounce/1
  Signal Conversion/1 -> Out/1  "Diag3_b1_TempIGBTFault_null"
  debounce/1 -> Signal Conversion/1

== system dgl_grc/Subsystem/OverTempDerare/IGBTTemp/Function-Call Subsystem/IGBTTempWarning ==
  note: % 85
  note: % -20
  note: % 20
  In1 : Inport
  In2 : Inport  Port=2
  In3 : Inport  Port=3
  Constant1 : Constant  Value=KDGL_TempIGBTWarningHeal_C  OutDataTypeStr=int16
  Constant2 : Constant  Value=KDGL_TempIGBTWarningErr_C  OutDataTypeStr=int16
  Logical Operator : Logic  Operator=OR  Inputs=3  AllPortsSameDT=off  OutDataTypeStr=boolean
  Relational Operator : RelationalOperator  OutDataTypeStr=boolean  InputSameDT=off
  Relational Operator1 : RelationalOperator  OutDataTypeStr=boolean  InputSameDT=off
  Relational Operator2 : RelationalOperator  OutDataTypeStr=boolean  InputSameDT=off
  Signal Conversion : SignalConversion  OverrideOpt=off
  T1 : Constant  Value=KDGL_IGBTStartDerat_C  OutDataTypeStr=single
  debounce : Library/debounce  SystemSampleTime=-1  VariantActivationTime=update diagram  AllowFlexibleInterface=on  Latency=0  AutoFrameSizeCalculation=off
  Out1 : Outport  VectorParamsAs1DForOutWhenUnconnected=off
  wires:
  In1/1 -> Relational Operator/1
  T1/1 -> Relational Operator2/2, Relational Operator1/2, Relational Operator/2
  In2/1 -> Relational Operator1/1
  In3/1 -> Relational Operator2/1
  Constant1/1 -> debounce/2
  Constant2/1 -> debounce/3
  Relational Operator/1 -> Logical Operator/1
  Relational Operator2/1 -> Logical Operator/3
  Relational Operator1/1 -> Logical Operator/2
  Logical Operator/1 -> debounce/1
  Signal Conversion/1 -> Out1/1  "Diag3_b1_TempIGBTWarning_null"
  debounce/1 -> Signal Conversion/1

== stateflow chart dgl_grc/Subsystem/OverLowVolDerate/HVLowMonitor/Chart ==
  note: %继电器闭合&&不是主动放电状态
  (default) -> (junction 6)
  (junction 6) -> (junction 4) [order 1] : [(BMS_bContactorClsd>=1)&&(ModControl~=6)]
  (junction 6) -> (junction 10) [order 2]
  (junction 4) -> (junction 7) : {
      | event;
      | }
  (junction 7) -> (junction 10)
  (junction 10) -> (junction 13)
  data: BMS_bContactorClsd input boolean; ModControl input uint8
  events: event output FUNCTION_CALL_EVENT
